simulink model "PMSMmotor_If"  (Simulink 8.9)
settings: Solver=ode45  StartTime=0  StopTime=2  FixedStep=1/fs/4  MaxStep=1/fs  RelTol=1e-7  EnableMultiTasking=on
undefined symbols (not defined in the file or in its folder): DiscIntNeverNeededParam, fs, Iphmax, J, Ki2, Ki3, Kp2, Kp3, Ld, Lndd_ini, Lndmpm, Lq, Npp, Omegae_ini, Rs, sigbuilder_block, Vph
libraries: simulink x1
settings Model: Creator=klu  LastModifiedBy=Martin
settings OptimizationCC: BooleanDataType=off  ExpressionDepthLimit=2147483647  InitFltsAndDblsToZero=on
settings DebuggingCC: AlgebraicLoopMsg=none  SaveWithParameterizedLinksMsg=none  SignalResolutionControl=TryResolveAllWithWarning  MultiTaskDSMMsg=warning  MultiTaskCondExecSysMsg=none
settings GRTTargetCC: TargetFcnLib=ansi_tfl_tmw.mat
settings ConfigComp: CovSFcnEnable=off

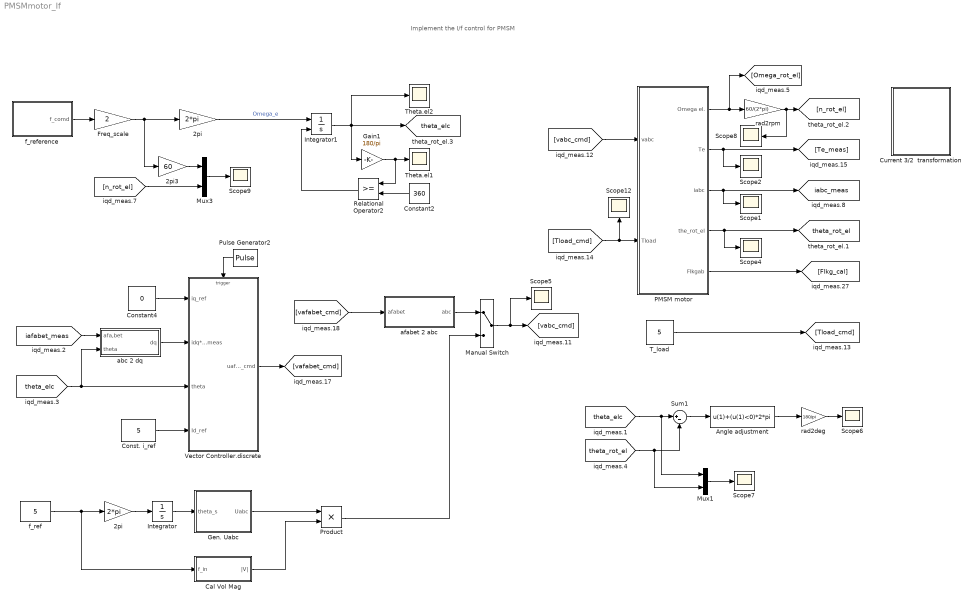
== system PMSMmotor_If ==
  note: Implement the I/f control for PMSM
  2pi : Gain  Gain=2*pi
  "2pi " : Gain  Gain=2*pi
  2pi3 : Gain  Gain=60
  Angle adjustment : Fcn  Expr=u(1)+(u(1)<0)*2*pi
  Cal Vol Mag : Subsystem
  Const. i_ref : Constant  Value=5
  Constant2 : Constant  Value=360
  Constant4 : Constant  Value=0
  Current 3/2  transformation : Subsystem
      mask Display:
      | plot([0.1000    0.1357    0.1714    0.2071    0.2429    0.2786    0.3143    0.3500    0.3857    0.4214 0.4571    0.4929    0.5286    0.5643    0.6000]-0.05,0.4+0.6*[0.5000    0.5868    0.6564    0.6950    0.6950    0.6564    0.5868    0.5000    0.4132    0.3436 0.3050    0.3050    0.3436    0.4132    0.5000])
      | 
      | plot([0.1,0.9],[0.1,0.9])
      | 
      | plot([0.5,0.9],0.3*[1 1])
  Freq_scale : Gain  Gain=2
  Gain1 : Gain  Gain=180/pi
  Gen. Uabc : Subsystem
  Integrator : Integrator
  Integrator1 : Integrator  ExternalReset=rising
  Manual Switch : ManualSwitch
  Mux1 : Mux  Inputs=2
  Mux3 : Mux  Inputs=2
  PMSM motor : Subsystem
  Product : Product  RndMeth=Zero
  Pulse Generator2 : DiscretePulseGenerator  PulseType=Time based  Period=1/fs  PulseWidth=50
  Relational Operator2 : RelationalOperator  OutDataTypeStr=boolean  RndMeth=Nearest
  Scope{1..2,4..9,12} (9 alike) : Scope
  Sum1 : Sum  Inputs=|+-
  T_load : Constant  Value=5
  Theta.el1 : Scope
  Theta.el2 : Scope
  Vector Controller.discrete : Subsystem
  abc 2 dq : Subsystem
  afabet 2 abc : Subsystem
  f_ref : Constant  Value=5
  f_reference : Subsystem  Tag=STV Subsys  LoadFcn=sigbuilder_block('load');  StartFcn=sigbuilder_block('start');  StopFcn=sigbuilder_block('stop');  ClipboardFcn=sigbuilder_block('clipboard');  mask(Sigbuilder block){tuvar=[0:10]}
      mask help: Simulink:masks:SigbuilderBlock_MD
      mask init:
      | if ~strcmp(get_param(bdroot(gcbh),'SimulationStatus'),'stopped') tuvar = sigbuilder_block('maskInit'); end
      settings: CopyFcn=sigbuilder_block('copy');  DeleteFcn=sigbuilder_block('delete');  ModelCloseFcn=sigbuilder_block('modelClose');  PreSaveFcn=sigbuilder_block('preSave');  PauseFcn=sigbuilder_block('pause');  ContinueFcn=sigbuilder_block('continue');  NameChangeFcn=sigbuilder_block('namechange');  OpenFcn=sigbuilder_block('open',[211.5 117.75 550.5 395.25 ]);  CloseFcn=sigbuilder_block('close');
      mask Display: plot(0, 0, 100, 100,[2, 2, 32, 32, 2], [68, 8, 8, 68, 68],[32, 2], [38, 38], [32, 19, 2],[53, 60, 44], [32, 17, 17, 2],[16, 16, 31, 31]);txt = getActiveGroup(gcbh);text(2, 100, txt,'verticalAlignment', 'top');
  rad2deg : Gain  Gain=180/pi
  rad2rpm : Gain  Gain=60/(2*pi)
  tag scope: iabc_meas=global, theta_elc=global, theta_rot_el=global
  wires:
  [Tload_cmd] -> PMSM motor/2(Tload), Scope12/1
  PMSM motor/2(Te) -> [Te_meas], Scope2/1
  PMSM motor/1(Omega el.) -> [Omega_rot_el], rad2rpm/1
  PMSM motor/3(iabc) -> Scope1/1, [iabc_meas]
  PMSM motor/4(the_rot_el) -> [theta_rot_el], Scope4/1
  [vabc_cmd] -> PMSM motor/1(vabc)
  Vector Controller.discrete/1(uafabet_cmd) -> [vafabet_cmd]
  [vafabet_cmd] -> afabet 2 abc/1(afabet)
  Pulse Generator2/1 -> Vector Controller.discrete/Trigger
  Const. i_ref/1 -> Vector Controller.discrete/4(Id_ref)
  PMSM motor/5(Flkgab) -> [Flkg_cal]
  [theta_elc] -> Vector Controller.discrete/3(theta), abc 2 dq/2(theta)
  f_reference/1(f_comd) -> Freq_scale/1
  Freq_scale/1 -> 2pi/1, 2pi3/1
  [iafabet_meas] -> abc 2 dq/1(afa,bet)
  abc 2 dq/1(dq) -> Vector Controller.discrete/2(idq*_meas)
  Integrator1/1 -> Theta.el2/1, Gain1/1, [theta_elc]
  Gain1/1 -> Theta.el1/1, Relational Operator2/1
  Constant2/1 -> Relational Operator2/2
  Relational Operator2/1 -> Integrator1/2
  2pi/1 -> Integrator1/1  "Omega_e"
  [theta_elc] -> Mux1/1, Sum1/1
  [theta_rot_el] -> Mux1/2, Sum1/2
  Sum1/1 -> Angle adjustment/1
  Angle adjustment/1 -> rad2deg/1
  rad2deg/1 -> Scope6/1
  Constant4/1 -> Vector Controller.discrete/1(iq_ref)
  Mux1/1 -> Scope7/1
  Mux3/1 -> Scope9/1
  2pi3/1 -> Mux3/1
  [n_rot_el] -> Mux3/2
  T_load/1 -> [Tload_cmd]
  rad2rpm/1 -> Scope8/1, [n_rot_el]
  "2pi "/1 -> Integrator/1
  Integrator/1 -> Gen. Uabc/1(theta_s)
  Gen. Uabc/1(Uabc) -> Product/1
  f_ref/1 -> Cal Vol Mag/1(f_in), "2pi "/1
  Cal Vol Mag/1(|V|) -> Product/2
  afabet 2 abc/1(abc) -> Manual Switch/1
  Manual Switch/1 -> [vabc_cmd], Scope5/1
  Product/1 -> Manual Switch/2

== system PMSMmotor_If/Cal Vol Mag ==
  f_in : Inport
  Vol Magnitude : Gain  Gain=4
  |V| : Outport
  wires:
  f_in/1 -> Vol Magnitude/1
  Vol Magnitude/1 -> |V|/1

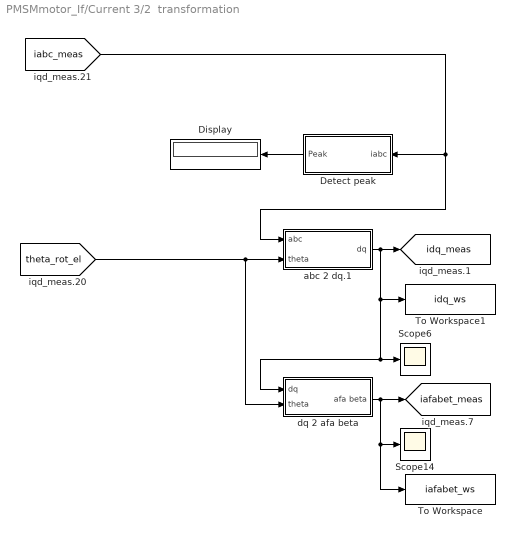
== system PMSMmotor_If/Current 3/2  transformation ==
  Detect peak : Subsystem
  Display : Display
  Scope14 : Scope
  Scope6 : Scope
  To Workspace : ToWorkspace  VariableName=iafabet_ws  SaveFormat=Structure With Time  SampleTime=1/fs/4
  To Workspace1 : ToWorkspace  VariableName=idq_ws  SaveFormat=Structure With Time  SampleTime=1/fs/4
  abc 2 dq.1 : Subsystem
  dq 2 afa beta : Subsystem
  tag scope: iafabet_meas=global, idq_meas=global
  wires:
  abc 2 dq.1/1(dq) -> [idq_meas], Scope6/1, dq 2 afa beta/1(dq), To Workspace1/1
  dq 2 afa beta/1(afa beta) -> [iafabet_meas], To Workspace/1, Scope14/1
  [iabc_meas] -> abc 2 dq.1/1(abc), Detect peak/1(iabc)
  Detect peak/1(Peak) -> Display/1
  [theta_rot_el] -> abc 2 dq.1/2(theta), dq 2 afa beta/2(theta)

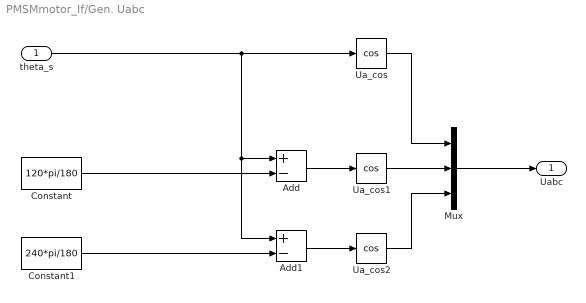
== system PMSMmotor_If/Gen. Uabc ==
  theta_s : Inport
  Add : Sum  Inputs=+-
  Add1 : Sum  Inputs=+-
  Constant : Constant  Value=120*pi/180
  Constant1 : Constant  Value=240*pi/180
  Mux : Mux  Inputs=3
  Ua_cos : Trigonometry  Operator=cos
  Ua_cos1 : Trigonometry  Operator=cos
  Ua_cos2 : Trigonometry  Operator=cos
  Uabc : Outport
  wires:
  Constant/1 -> Add/2
  Constant1/1 -> Add1/2
  theta_s/1 -> Ua_cos/1, Add/1, Add1/1
  Add/1 -> Ua_cos1/1
  Add1/1 -> Ua_cos2/1
  Ua_cos/1 -> Mux/1
  Ua_cos1/1 -> Mux/2
  Ua_cos2/1 -> Mux/3
  Mux/1 -> Uabc/1

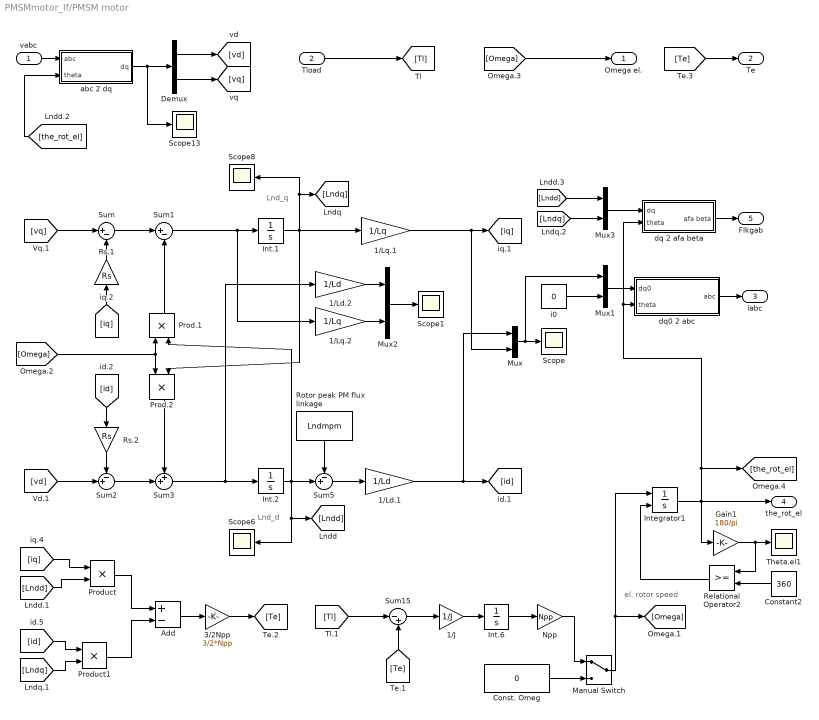
== system PMSMmotor_If/PMSM motor ==
  note: Lnd_d
  note: Lnd_q
  note: el. rotor speed
  vabc : Inport
  Tload : Inport  Port=2
  1/J : Gain  Gain=1/J
  1/Ld.1 : Gain  Gain=1/Ld
  1/Ld.2 : Gain  Gain=1/Ld
  1/Lq.1 : Gain  Gain=1/Lq
  1/Lq.2 : Gain  Gain=1/Lq
  3/2Npp : Gain  Gain=3/2*Npp
  Add : Sum  Inputs=+-
  Const. Omeg : Constant  Value=0
  Constant2 : Constant  Value=360
  Demux : Demux  Outputs=2
  Gain1 : Gain  Gain=180/pi
  Int.1 : Integrator
  Int.2 : Integrator  InitialCondition=Lndd_ini
  Int.6 : Integrator  InitialCondition=Omegae_ini/Npp
  Integrator1 : Integrator  ExternalReset=rising
  Manual Switch : ManualSwitch
  Mux{,1..3} (4 alike) : Mux  Inputs=2
  Npp : Gain  Gain=Npp
  Prod.1 : Product  RndMeth=Zero
  Prod.2 : Product  RndMeth=Zero
  Product : Product  RndMeth=Zero
  Product1 : Product  RndMeth=Zero
  Relational Operator2 : RelationalOperator  OutDataTypeStr=boolean  RndMeth=Nearest
  Rotor peak PM flux linkage : Constant  Value=Lndmpm
  Rs.1 : Gain  Gain=Rs
  Rs.2 : Gain  Gain=Rs
  Scope{,1,6,8,13} (5 alike) : Scope
  Sum : Sum  Inputs=|+-
  Sum1 : Sum  Inputs=|+-
  Sum15 : Sum  Inputs=|-+
  Sum2 : Sum  Inputs=-+|
  Sum3 : Sum  Inputs=++|
  Sum5 : Sum  Inputs=-+|
  Theta.el1 : Scope
  abc 2 dq : Subsystem
  dq 2 afa beta : Subsystem
  dq0 2 abc : Subsystem
  i0 : Constant  Value=0
  Omega el. : Outport
  Te : Outport  Port=2
  iabc : Outport  Port=3
  the_rot_el : Outport  Port=4
  Flkgab : Outport  Port=5
  wires:
  3/2Npp/1 -> [Te]
  Add/1 -> 3/2Npp/1
  Sum5/1 -> 1/Ld.1/1
  Rotor peak PM flux linkage/1 -> Sum5/1
  [Omega] -> Omega el./1
  [Te] -> Te/1
  Product1/1 -> Add/2
  Product/1 -> Add/1
  [Lndq] -> Product1/2
  [id] -> Product1/1
  [Lndd] -> Product/2
  [iq] -> Product/1
  [Te] -> Sum15/2
  Int.6/1 -> Npp/1
  1/J/1 -> Int.6/1
  Sum15/1 -> 1/J/1
  [Tl] -> Sum15/1
  Mux/1 -> Scope/1, Mux1/1
  [Omega] -> Prod.2/1, Prod.1/1
  Sum3/1 -> Int.2/1, 1/Ld.2/1
  Prod.2/1 -> Sum3/1
  Sum2/1 -> Sum3/2
  [id] -> Rs.2/1
  Rs.2/1 -> Sum2/1
  [vd] -> Sum2/2
  1/Ld.1/1 -> [id], Mux/1
  Int.2/1 -> Scope6/1, [Lndd], Sum5/2, Prod.1/2
  [iq] -> Rs.1/1
  1/Lq.1/1 -> [iq], Mux/2
  Prod.1/1 -> Sum1/2
  Sum1/1 -> Int.1/1, 1/Lq.2/1
  Int.1/1 -> 1/Lq.1/1, Prod.2/2, Scope8/1, [Lndq]
  Sum/1 -> Sum1/1
  Rs.1/1 -> Sum/2
  [vq] -> Sum/1
  Tload/1 -> [Tl]
  Demux/2 -> [vq]
  Demux/1 -> [vd]
  i0/1 -> Mux1/2
  Mux1/1 -> dq0 2 abc/1(dq0)
  dq0 2 abc/1(abc) -> iabc/1
  Integrator1/1 -> Gain1/1, the_rot_el/1, dq 2 afa beta/2(theta), dq0 2 abc/2(theta), [the_rot_el]
  Gain1/1 -> Theta.el1/1, Relational Operator2/1
  Constant2/1 -> Relational Operator2/2
  Relational Operator2/1 -> Integrator1/2
  vabc/1 -> abc 2 dq/1(abc)
  abc 2 dq/1(dq) -> Demux/1, Scope13/1
  [the_rot_el] -> abc 2 dq/2(theta)
  Const. Omeg/1 -> Manual Switch/2
  Manual Switch/1 -> [Omega], Integrator1/1
  Npp/1 -> Manual Switch/1
  1/Ld.2/1 -> Mux2/1
  1/Lq.2/1 -> Mux2/2
  Mux2/1 -> Scope1/1
  Mux3/1 -> dq 2 afa beta/1(dq)
  [Lndd] -> Mux3/1
  [Lndq] -> Mux3/2
  dq 2 afa beta/1(afa beta) -> Flkgab/1

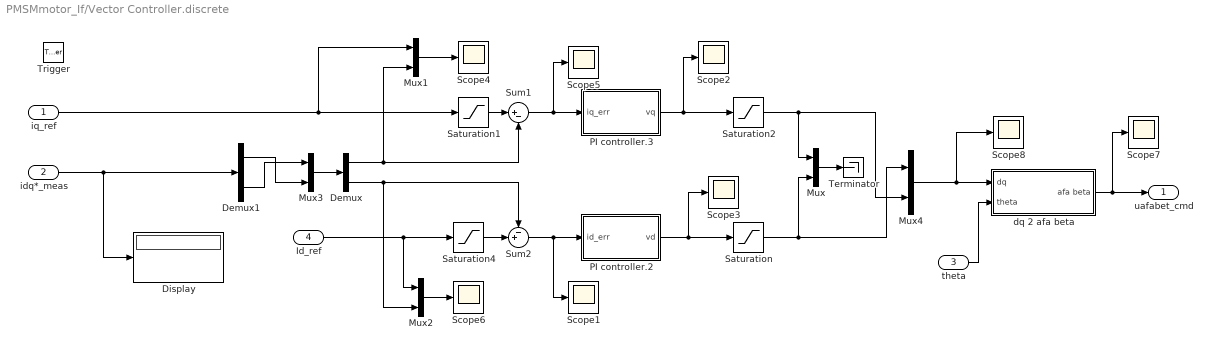
== system PMSMmotor_If/Vector Controller.discrete ==
  iq_ref : Inport
  idq*_meas : Inport  Port=2
  theta : Inport  Port=3
  Id_ref : Inport  Port=4
  Trigger : TriggerPort  VariantControl=Variant
  Demux : Demux  Outputs=2
  Demux1 : Demux  Outputs=2
  Display : Display
  Mux{,1..4} (5 alike) : Mux  Inputs=2
  PI controller.2 : Subsystem
  PI controller.3 : Subsystem
  Saturation : Saturate  UpperLimit=Vph  LowerLimit=-Vph
  Saturation1 : Saturate  UpperLimit=Iphmax  LowerLimit=-Iphmax
  Saturation2 : Saturate  UpperLimit=Vph  LowerLimit=-Vph
  Saturation4 : Saturate  UpperLimit=Iphmax  LowerLimit=-Iphmax
  Scope{1..8} (8 alike) : Scope
  Sum1 : Sum  Inputs=|+-
  Sum2 : Sum  Inputs=-+|
  Terminator : Terminator
  dq 2 afa beta : Subsystem
  uafabet_cmd : Outport
  wires:
  Saturation4/1 -> Sum2/2
  Saturation/1 -> Mux/2, Mux4/1
  Mux/1 -> Terminator/1
  PI controller.3/1(vq) -> Scope2/1, Saturation2/1
  Demux/1 -> Sum1/2, Mux1/2
  PI controller.2/1(vd) -> Saturation/1, Scope3/1
  Demux/2 -> Sum2/1, Mux2/2
  Sum1/1 -> Scope5/1, PI controller.3/1(iq_err)
  iq_ref/1 -> Mux1/1, Saturation1/1
  Sum2/1 -> Scope1/1, PI controller.2/1(id_err)
  Id_ref/1 -> Saturation4/1, Mux2/1
  Mux1/1 -> Scope4/1
  Saturation1/1 -> Sum1/1
  Mux2/1 -> Scope6/1
  Saturation2/1 -> Mux4/2, Mux/1
  Mux4/1 -> Scope8/1, dq 2 afa beta/1(dq)
  Mux3/1 -> Demux/1
  idq*_meas/1 -> Display/1, Demux1/1
  dq 2 afa beta/1(afa beta) -> Scope7/1, uafabet_cmd/1
  theta/1 -> dq 2 afa beta/2(theta)
  Demux1/1 -> Mux3/2
  Demux1/2 -> Mux3/1

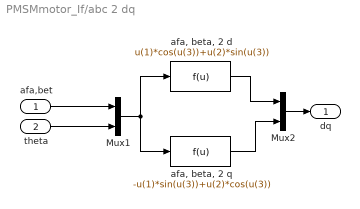
== system PMSMmotor_If/abc 2 dq ==
  afa,bet : Inport
  theta : Inport  Port=2
  Mux1 : Mux  Inputs=2
  Mux2 : Mux  Inputs=2
  "afa, beta, 2 d" : Fcn  Expr=u(1)*cos(u(3))+u(2)*sin(u(3))
  "afa, beta, 2 q" : Fcn  Expr=-u(1)*sin(u(3))+u(2)*cos(u(3))
  dq : Outport
  wires:
  Mux2/1 -> dq/1
  "afa, beta, 2 q"/1 -> Mux2/2
  "afa, beta, 2 d"/1 -> Mux2/1
  Mux1/1 -> "afa, beta, 2 q"/1, "afa, beta, 2 d"/1
  theta/1 -> Mux1/2
  afa,bet/1 -> Mux1/1

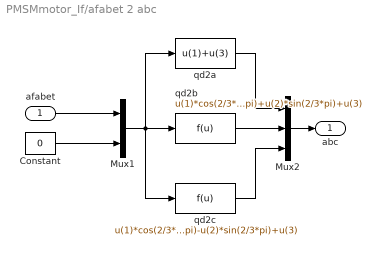
== system PMSMmotor_If/afabet 2 abc ==
  afabet : Inport
  Constant : Constant  Value=0
  Mux1 : Mux  Inputs=2
  Mux2 : Mux  Inputs=3
  qd2a : Fcn  Expr=u(1)+u(3)
  qd2b : Fcn  Expr=u(1)*cos(2/3*pi)+u(2)*sin(2/3*pi)+u(3)
  qd2c : Fcn  Expr=u(1)*cos(2/3*pi)-u(2)*sin(2/3*pi)+u(3)
  abc : Outport
  wires:
  Constant/1 -> Mux1/2
  qd2c/1 -> Mux2/3
  afabet/1 -> Mux1/1
  Mux1/1 -> qd2c/1, qd2b/1, qd2a/1
  qd2a/1 -> Mux2/1
  qd2b/1 -> Mux2/2
  Mux2/1 -> abc/1

== system PMSMmotor_If/f_reference ==
  Demux : Demux  Tag=STV Demux  Outputs=1
  FromWs : FromWorkspace  Tag=STV FromWs  VariableName=tuvar  SampleTime=0  SigBuilderData=DataTag0  VnvData=DataTag1
      SigBuilderData=|
      | common.afterFinalStr = 'Extrapolate'
      | common.sampleTime = 0
      | dataSet.timeRange = [0 10]
      | dataSet.name = 'Group 1'
      | sbobj.Groups.Name = 'Group 1'
      | sbobj.Groups.Signals.Name = 'f_comd'
      | sbobj.Groups.Signals.XData = [0 1 2 10]
      | sbobj.Groups.Signals.YData = [0 1 1 1]
  f_comd : Outport  Tag=STV Outport
  wires:
  FromWs/1 -> Demux/1
  Demux/1 -> f_comd/1

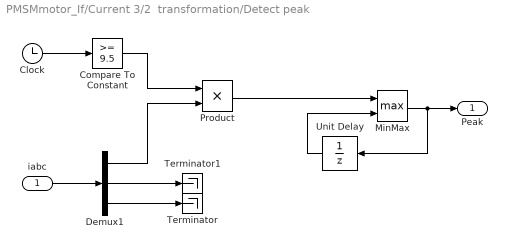
== system PMSMmotor_If/Current 3/2  transformation/Detect peak ==
  iabc : Inport
  Clock : Clock
  Compare To Constant : simulink/Logic and Bit Operations/Compare To Constant  relop=>=  const=9.5  OutDataTypeStr=uint8  ZeroCross=off
  Demux1 : Demux  Outputs=3
  MinMax : MinMax  Function=max  Inputs=2
  Product : Product  RndMeth=Zero
  Terminator : Terminator
  Terminator1 : Terminator
  Unit Delay : UnitDelay  SampleTime=1/5e3
  Peak : Outport
  wires:
  iabc/1 -> Demux1/1
  Demux1/3 -> Terminator/1
  Demux1/2 -> Terminator1/1
  Clock/1 -> Compare To Constant/1
  Compare To Constant/1 -> Product/1
  Demux1/1 -> Product/2
  MinMax/1 -> Peak/1, Unit Delay/1
  Product/1 -> MinMax/1
  Unit Delay/1 -> MinMax/2

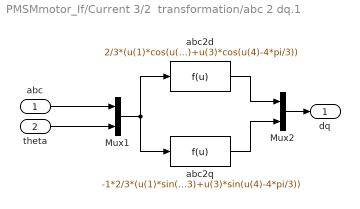
== system PMSMmotor_If/Current 3/2  transformation/abc 2 dq.1 ==
  abc : Inport
  theta : Inport  Port=2
  Mux1 : Mux  Inputs=2
  Mux2 : Mux  Inputs=2
  abc2d : Fcn  Expr=2/3*(u(1)*cos(u(4))+u(2)*cos(u(4)-2*pi/3)+u(3)*cos(u(4)-4*pi/3))
  abc2q : Fcn  Expr=-1*2/3*(u(1)*sin(u(4))+u(2)*sin(u(4)-2*pi/3)+u(3)*sin(u(4)-4*pi/3))
  dq : Outport
  wires:
  Mux2/1 -> dq/1
  abc2q/1 -> Mux2/2
  abc2d/1 -> Mux2/1
  Mux1/1 -> abc2q/1, abc2d/1
  theta/1 -> Mux1/2
  abc/1 -> Mux1/1

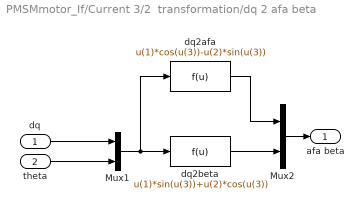
== system PMSMmotor_If/Current 3/2  transformation/dq 2 afa beta ==
  dq : Inport
  theta : Inport  Port=2
  Mux1 : Mux  Inputs=2
  Mux2 : Mux  Inputs=2
  dq2afa : Fcn  Expr=u(1)*cos(u(3))-u(2)*sin(u(3))
  dq2beta : Fcn  Expr=u(1)*sin(u(3))+u(2)*cos(u(3))
  afa beta : Outport
  wires:
  dq/1 -> Mux1/1
  theta/1 -> Mux1/2
  Mux1/1 -> dq2beta/1, dq2afa/1
  dq2afa/1 -> Mux2/1
  dq2beta/1 -> Mux2/2
  Mux2/1 -> afa beta/1

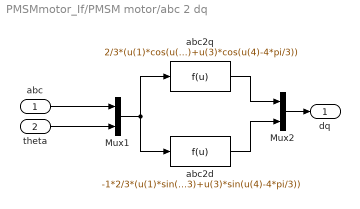
== system PMSMmotor_If/PMSM motor/abc 2 dq ==
  abc : Inport
  theta : Inport  Port=2
  Mux1 : Mux  Inputs=2
  Mux2 : Mux  Inputs=2
  abc2d : Fcn  Expr=-1*2/3*(u(1)*sin(u(4))+u(2)*sin(u(4)-2*pi/3)+u(3)*sin(u(4)-4*pi/3))
  abc2q : Fcn  Expr=2/3*(u(1)*cos(u(4))+u(2)*cos(u(4)-2*pi/3)+u(3)*cos(u(4)-4*pi/3))
  dq : Outport
  wires:
  Mux2/1 -> dq/1
  abc2d/1 -> Mux2/2
  abc2q/1 -> Mux2/1
  Mux1/1 -> abc2d/1, abc2q/1
  theta/1 -> Mux1/2
  abc/1 -> Mux1/1

== system PMSMmotor_If/PMSM motor/dq 2 afa beta ==
  dq : Inport
  theta : Inport  Port=2
  Mux1 : Mux  Inputs=2
  Mux2 : Mux  Inputs=2
  dq2afa : Fcn  Expr=u(1)*cos(u(3))-u(2)*sin(u(3))
  dq2beta : Fcn  Expr=u(1)*sin(u(3))+u(2)*cos(u(3))
  afa beta : Outport
  wires:
  dq/1 -> Mux1/1
  theta/1 -> Mux1/2
  Mux1/1 -> dq2beta/1, dq2afa/1
  dq2afa/1 -> Mux2/1
  dq2beta/1 -> Mux2/2
  Mux2/1 -> afa beta/1

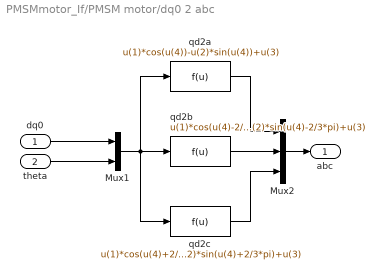
== system PMSMmotor_If/PMSM motor/dq0 2 abc ==
  dq0 : Inport
  theta : Inport  Port=2
  Mux1 : Mux  Inputs=2
  Mux2 : Mux  Inputs=3
  qd2a : Fcn  Expr=u(1)*cos(u(4))-u(2)*sin(u(4))+u(3)
  qd2b : Fcn  Expr=u(1)*cos(u(4)-2/3*pi)-u(2)*sin(u(4)-2/3*pi)+u(3)
  qd2c : Fcn  Expr=u(1)*cos(u(4)+2/3*pi)-u(2)*sin(u(4)+2/3*pi)+u(3)
  abc : Outport
  wires:
  Mux2/1 -> abc/1
  qd2b/1 -> Mux2/2
  qd2a/1 -> Mux2/1
  Mux1/1 -> qd2a/1, qd2b/1, qd2c/1
  theta/1 -> Mux1/2
  dq0/1 -> Mux1/1
  qd2c/1 -> Mux2/3

== system PMSMmotor_If/Vector Controller.discrete/PI controller.2 ==
  id_err : Inport
  Discrete-Time Integrator : DiscreteIntegrator  SampleTime=-1  ICPrevOutput=DiscIntNeverNeededParam  ICPrevScaledInput=DiscIntNeverNeededParam
  Kp : Gain  Gain=Kp2
  Sum1 : Sum  Inputs=|++
  ki : Gain  Gain=Ki2
  vd : Outport
  wires:
  Sum1/1 -> vd/1
  Discrete-Time Integrator/1 -> Sum1/2
  ki/1 -> Discrete-Time Integrator/1
  Kp/1 -> Sum1/1
  id_err/1 -> ki/1, Kp/1

== system PMSMmotor_If/Vector Controller.discrete/PI controller.3 ==
  iq_err : Inport
  Discrete-Time Integrator : DiscreteIntegrator  SampleTime=-1  ICPrevOutput=DiscIntNeverNeededParam  ICPrevScaledInput=DiscIntNeverNeededParam
  Kp : Gain  Gain=Kp3
  Sum1 : Sum  Inputs=|++
  ki : Gain  Gain=Ki3
  vq : Outport
  wires:
  Sum1/1 -> vq/1
  Discrete-Time Integrator/1 -> Sum1/2
  ki/1 -> Discrete-Time Integrator/1
  Kp/1 -> Sum1/1
  iq_err/1 -> ki/1, Kp/1

== system PMSMmotor_If/Vector Controller.discrete/dq 2 afa beta ==
  dq : Inport
  theta : Inport  Port=2
  Mux1 : Mux  Inputs=2
  Mux2 : Mux  Inputs=2
  dq2afa : Fcn  Expr=u(1)*cos(u(3))-u(2)*sin(u(3))
  dq2beta : Fcn  Expr=u(1)*sin(u(3))+u(2)*cos(u(3))
  afa beta : Outport
  wires:
  Mux2/1 -> afa beta/1
  dq2beta/1 -> Mux2/2
  dq2afa/1 -> Mux2/1
  Mux1/1 -> dq2afa/1, dq2beta/1
  theta/1 -> Mux1/2
  dq/1 -> Mux1/1
